simulink model "proyecto_2"  (R2021b)
settings: Solver=FixedStepDiscrete  StartTime=0.0  StopTime=Tsim  FixedStep=Tint  MaxStep=1e-6  RelTol=1e-6
InitFcn:
  | run init_fcn.m;
values from neighbouring files (symbols this model uses):
  C_init_v = 317    [init_fcn.m]
  C_load = 5e-2    (= 0.05)    [init_fcn.m]
  C_V = c_v * ro_air * volume_room    (= 220.63309632)    [init_fcn.m]
  Irr = 1000    [init_fcn.m]
  K_cond = Window_area * k_glass / esp    (= 158.4)    [init_fcn.m]
  L_s = 5e-3    (= 0.005)    [init_fcn.m]
  R_cuarto = 100    [init_fcn.m]
  shift = (180/3)/360 * Ts    (= 8.33333333333e-05)    [init_fcn.m]
  ss2 = c2d(ss2c, T_pred, 'tustin')    [init_fcn.m]
  T_ext = 15    [init_fcn.m]
  T_pred = Ts    (= 0.0005)    [init_fcn.m]
  Tint = 5e-5    (= 5e-05)    [init_fcn.m]
  Ts = 0.0005    [init_fcn.m]
  V_H4 = 300    [init_fcn.m]
  V_source = 230 * sqrt(2)    [init_fcn.m]
undefined symbols (not defined in the file or in its folder): DiscIntNeverNeededParam, F, K, Kobs, M, N, N2, Q, T_Enable, Temp_ref, Tsim, U0, X0
libraries: spsIGBTDiodeLib x17, spsVoltageMeasurementLib x11, simulink x8, spsCurrentMeasurementLib x8, slpidlib x6, spsSeriesRLCBranchLib x5, spsParallelRLCBranchLib x4, spsPVArrayLib x3, spsACVoltageSourceLib x1, spsDiodeLib x1, spspowerguiLib x1
(part 1 of 2)
settings Model: Creator=david  LastModifiedBy=david
settings DebuggingCC: UnderSpecifiedDimensionMsg=warning

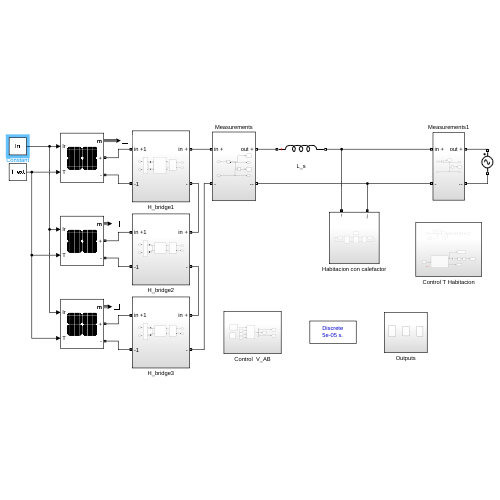
[thumbnail: Simulink's stored preview of the top-level diagram]
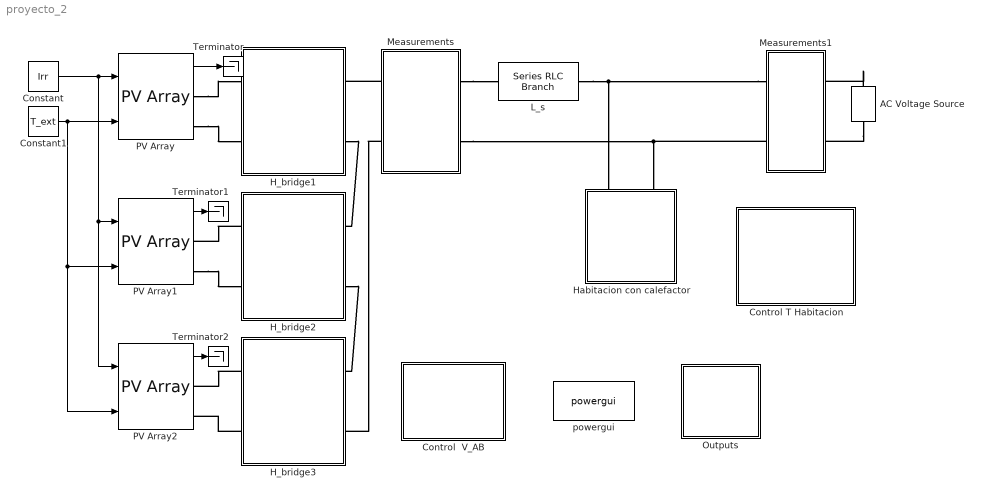
== system proyecto_2 ==
  AC Voltage Source : spsACVoltageSourceLib/AC Voltage Source  Amplitude=V_source  Phase=0  Frequency=50  SampleTime=0  Measurements=None  BusType=swing  Pref=10e3  Qref=0  Qmin=-inf  Qmax=+inf
  Constant : Constant  Value=Irr
  Constant1 : Constant  Value=T_ext
  Control  V_AB : Subsystem
  Control T Habitacion : Subsystem
  H_bridge1 : Subsystem
  H_bridge2 : Subsystem
  H_bridge3 : Subsystem
  Habitacion con calefactor : Subsystem
  L_s : spsSeriesRLCBranchLib/Series RLC Branch  LConnTagsString=__new0  RConnTagsString=__new0  BranchType=L  Resistance=1  Inductance=L_s*5  SetiL0=off  InitialCurrent=0  Capacitance=1e-6  Setx0=off  InitialVoltage=0  Measurements=None
  Measurements : Subsystem
  Measurements1 : Subsystem
  Outputs : Subsystem
  PV Array : spsPVArrayLib/PV Array  Npar=1  Nser=10  PlotType=array @ 1000 W/m2 & specified temperatures  S_vec="[ 1000  500  100 ]"  Temp_C_vec="[ 45 25  ]"  ModuleName=Ablytek 6PN6A230-A0  PlotWhenSelected=off  Pm=230.1288  Ncell=60  Voc=36.42  Isc=8.1  Vm=30.36  Im=7.58  beta_Voc_pc=-0.359  alpha_Isc_pc=0.097  beta_Voc=-0.13075  alpha_Isc=0.007857  IL=8.1068  I0=2.7914e-10  nI=0.98144  Rsh=234.4444  Rs=0.19819  RobustModel=off  RobustCellTemperature=313.3991  BAL=on  Tc=1e-6  Tfilter=5e-5
  PV Array1 : spsPVArrayLib/PV Array  Npar=1  Nser=10  PlotType=array @ 1000 W/m2 & specified temperatures  S_vec="[ 1000  500  100 ]"  Temp_C_vec="[ 45 25  ]"  ModuleName=Ablytek 6PN6A230-A0  PlotWhenSelected=off  Pm=230.1288  Ncell=60  Voc=36.42  Isc=8.1  Vm=30.36  Im=7.58  beta_Voc_pc=-0.359  alpha_Isc_pc=0.097  beta_Voc=-0.13075  alpha_Isc=0.007857  IL=8.1068  I0=2.7914e-10  nI=0.98144  Rsh=234.4444  Rs=0.19819  RobustModel=off  RobustCellTemperature=313.3991  BAL=on  Tc=1e-6  Tfilter=5e-5
  PV Array2 : spsPVArrayLib/PV Array  Npar=1  Nser=10  PlotType=array @ 1000 W/m2 & specified temperatures  S_vec="[ 1000  500  100 ]"  Temp_C_vec="[ 45 25  ]"  ModuleName=Ablytek 6PN6A230-A0  PlotWhenSelected=off  Pm=230.1288  Ncell=60  Voc=36.42  Isc=8.1  Vm=30.36  Im=7.58  beta_Voc_pc=-0.359  alpha_Isc_pc=0.097  beta_Voc=-0.13075  alpha_Isc=0.007857  IL=8.1068  I0=2.7914e-10  nI=0.98144  Rsh=234.4444  Rs=0.19819  RobustModel=off  RobustCellTemperature=313.3991  BAL=on  Tc=1e-6  Tfilter=5e-5
  Terminator : Terminator
  Terminator1 : Terminator
  Terminator2 : Terminator
  powergui : spspowerguiLib/powergui  Priority=1  SimulationMode=Discrete  SampleTime=Tint  frequency=60  Iterations=50  frequencyindice=0  Pbase=100e6  ErrMax=1e-4  UnitsV=kV  UnitsW=MW  buscounter=0  FunctionMessages=off  echomessages=off  EnableUseOfTLC=off  CurrentSourceSwitches=off  DisableSnubberDevices=off  DisableRonSwitches=off  DisableVfSwitches=off  DisplayEquations=off  AutomaticDiscreteSolvers=off  SolverType=Tustin/Backward Euler (TBE)  Interpol=off  ExternalGateDelay=off  methode=off  Ts=100  x0status=blocks  SPID=on  SwTol=0  HookPort=off  NonlinearTolerance=1e-4  nMaxIteration=100  ContinueOnMaxIteration=off  RestoreLinks=warning  ResistiveCurrentMeasurement=off  Frange=[0:2:500]  Ylog=off  Xlog=on  ShowGrid=off  save=off  variable=ZData  structure=0  ZoomFFT=off  StartTime=0.0  cycles=1  DisplayStyle=1  fundamental=60  FreqAxis=off  MaxFrequency=1000  frequencyindicesteady=1  RmsSteady=1  display=off
  wires:
  Constant1/1 -> PV Array1/2, PV Array2/2, PV Array/2
  Constant/1 -> PV Array2/1, PV Array1/1, PV Array/1
  PV Array/1 -> Terminator/1
  PV Array1/1 -> Terminator1/1
  PV Array2/1 -> Terminator2/1
  connections:
  PV Array/RConn2 -- H_bridge1/LConn2
  PV Array/RConn1 -- H_bridge1/LConn1
  Measurements/LConn1 -- H_bridge1/RConn1
  Measurements/RConn1 -- L_s/LConn1
  Measurements1/LConn2 -- Measurements/RConn2 -- Habitacion con calefactor/LConn2
  AC Voltage Source/RConn1 -- Measurements1/RConn1
  AC Voltage Source/LConn1 -- Measurements1/RConn2
  H_bridge1/RConn2 -- H_bridge2/RConn1
  H_bridge3/LConn1 -- PV Array2/RConn1
  H_bridge2/RConn2 -- H_bridge3/RConn1
  Measurements/LConn2 -- H_bridge3/RConn2
  PV Array1/RConn2 -- H_bridge2/LConn2
  H_bridge2/LConn1 -- PV Array1/RConn1
  H_bridge3/LConn2 -- PV Array2/RConn2
  L_s/RConn1 -- Measurements1/LConn1 -- Habitacion con calefactor/LConn1

== system proyecto_2/Control  V_AB ==
  DC-bus control : Subsystem
  Demux1 : Demux  Outputs=3
  S-Function : S-Function  FunctionName=ff3dm  SFunctionDeploymentMode=off  EnableBusSupport=off
  reassignment : Subsystem
  tag scope: d_1=global, d_2=global, d_3=global
  wires:
  [I_ab] -> S-Function/2
  Demux1/1 -> [d_1]
  Demux1/2 -> [d_2]
  Demux1/3 -> [d_3]
  S-Function/1 -> Demux1/1
  [refs] -> S-Function/4
  [V_dcH] -> S-Function/3
  DC-bus control/1(Out1) -> S-Function/1

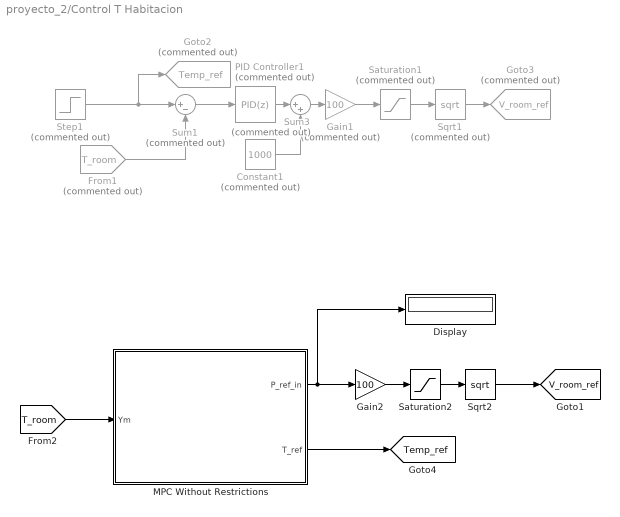
== system proyecto_2/Control T Habitacion ==
  Constant1 : Constant  Commented=on  Value=1000
  Display : Display
  From1 : From  Commented=on  GotoTag=T_room  TagVisibility=global
  Gain1 : Gain  Commented=on  Gain=100
  Gain2 : Gain  Gain=100
  Goto2 : Goto  Commented=on  GotoTag=Temp_ref  TagVisibility=global
  Goto3 : Goto  Commented=on  GotoTag=V_room_ref  TagVisibility=global
  MPC Without Restrictions : Subsystem
  PID Controller1 : slpidlib/PID Controller  Commented=on  Controller=PID  Form=Parallel  TimeDomain=Discrete-time  UseExternalTs=off  SampleTime=10*Ts  IntegratorMethod=Forward Euler  FilterMethod=Forward Euler  ControllerParametersSource=internal  P=200  I=500  D=0  UseFilter=on  N=100  TunerSelectOption=Transfer Function Based (PID Tuner App)  InitialConditionSource=internal  InitialConditionForIntegrator=0  InitialConditionForFilter=0  DifferentiatorICPrevScaledInput=0  ExternalReset=none  TrackingMode=off  Kt=1  LimitOutput=off  SatLimitsSource=internal  UpperSaturationLimit=inf  LowerSaturationLimit=-inf  LinearizeAsGain=on  AntiWindupMode=none  Kb=1  POutMin=[]  POutMax=[]  IOutMin=[]  IOutMax=[]  DOutMin=[]  DOutMax=[]  NOutMin=[]  NOutMax=[]  SumOutMin=[]  SumOutMax=[]  SaturationOutMin=[]  SaturationOutMax=[]  PParamMin=[]  PParamMax=[]  IParamMin=[]  IParamMax=[]  DParamMin=[]  DParamMax=[]  NParamMin=[]  NParamMax=[]  KbParamMin=[]  KbParamMax=[]  KtParamMin=[]  KtParamMax=[]  KbOutMin=[]  KbOutMax=[]  KtOutMin=[]  KtOutMax=[]  IntegratorOutMin=[]  IntegratorOutMax=[]  FilterOutMin=[]  FilterOutMax=[]  SumI1OutMin=[]  SumI1OutMax=[]  SumI2OutMin=[]  SumI2OutMax=[]  SumI3OutMin=[]  SumI3OutMax=[]  SumI4OutMin=[]  SumI4OutMax=[]  SumDOutMin=[]  SumDOutMax=[]  DifferentiatorOutMin=[]  DifferentiatorOutMax=[]  FilterDiffOutCoefMin=[]  FilterDiffOutCoefMax=[]  ReciprocalOutMin=[]  ReciprocalOutMax=[]  SumDenOutMin=[]  SumDenOutMax=[]  SumNumOutMin=[]  SumNumOutMax=[]  DivideOutMin=[]  DivideOutMax=[]  UdiffTsProdOutMin=[]  UdiffTsProdOutMax=[]  NTsProdOutMin=[]  NTsProdOutMax=[]  UintegralTsProdOutMin=[]  UintegralTsProdOutMax=[]  UngainTsProdOutMin=[]  UngainTsProdOutMax=[]  IntegratorContinuousStateAttributes=''  IntegratorStateMustResolveToSignalObject=off  IntegratorRTWStateStorageClass=Auto  FilterContinuousStateAttributes=''  FilterStateMustResolveToSignalObject=off  FilterRTWStateStorageClass=Auto  ParallelPVariant=InternalParameters  IdealPVariant=Disabled  IVariant=InternalParameters  DVariant=InternalParameters  IntegratorVariant=Discrete  SatVariant=Disabled  AWVariant=Passthrough  PCopyVariant=Disabled  TRVariant=Disabled  FdbkBlocksVariant=Forward  IdealPFdbkVariant=Disabled  SatFdbkVariant=Disabled  DerivativeFilterVariant=ForwardEulerFilter  NVariant=InternalParameters  NCopyVariant=Disabled  FilterICVariant=InternalICsFilter  IntegratorICVariant=InternalICs  ExternalResetVariant=Disabled  TRSumVariant=Passthrough  SumFdbkVariant=Disabled  SumVariant=Sum_PID  TsampFilterVariant=InternalTs  TsampNgainVariant=Passthrough  TsampIntegralVariant=Passthrough  ExternalSaturationOutDataTypeStr=Inherit: Same as second input
  Saturation1 : Saturate  Commented=on  UpperLimit=inf  LowerLimit=0
  Saturation2 : Saturate  UpperLimit=inf  LowerLimit=0
  Sqrt1 : Sqrt  Commented=on  SaturateOnIntegerOverflow=on
  Sqrt2 : Sqrt  SaturateOnIntegerOverflow=on
  Step1 : Step  Commented=on  Time=5  Before=20  After=25  SampleTime=0
  Sum1 : Sum  Commented=on  Inputs=|+-
  Sum3 : Sum  Commented=on  Inputs=|++
  tag scope: Temp_ref=global, V_room_ref=global
  wires:
  PID Controller1/1 -> Sum3/1
  Sum1/1 -> PID Controller1/1
  Constant1/1 -> Sum3/2
  Sqrt1/1 -> Goto3/1
  Gain1/1 -> Saturation1/1
  From1/1 -> Sum1/2
  Saturation1/1 -> Sqrt1/1
  Sum3/1 -> Gain1/1
  Step1/1 -> Goto2/1, Sum1/1
  Saturation2/1 -> Sqrt2/1
  Gain2/1 -> Saturation2/1
  MPC Without Restrictions/2(T_ref) -> [Temp_ref]
  MPC Without Restrictions/1(P_ref_in) -> Gain2/1, Display/1
  Sqrt2/1 -> [V_room_ref]
  [T_room] -> MPC Without Restrictions/1(Ym)
  ? -> ?

== system proyecto_2/H_bridge1 ==
  H_basic : Subsystem
  Measurements : Subsystem
  Measurements1 : Subsystem
  Parallel RLC Branch : spsParallelRLCBranchLib/Parallel RLC Branch  LConnTagsString=a  RConnTagsString=__new0  BranchType=C  Resistance=1  Inductance=1e-3  SetiL0=off  InitialCurrent=0  Capacitance=C_load  Setx0=on  InitialVoltage=C_init_v  Measurements=None
  in +1 : PMIOPort  Side=Left
  -1 : PMIOPort  Port=2  Side=Left
  in + : PMIOPort  Port=3  Side=Right
  - : PMIOPort  Port=4  Side=Right
  connections:
  Measurements1/RConn1 -- Parallel RLC Branch/LConn1 -- H_basic/LConn1
  Measurements/LConn1 -- in +/RConn1
  Measurements1/RConn2 -- Parallel RLC Branch/RConn1 -- H_basic/LConn2
  Measurements1/LConn1 -- in +1/RConn1
  Measurements1/LConn2 -- -1/RConn1
  Measurements/RConn2 -- H_basic/RConn2
  Measurements/LConn2 -- -/RConn1
  Measurements/RConn1 -- H_basic/RConn1

== system proyecto_2/H_bridge2 ==
  H_basic : Subsystem
  Measurements : Subsystem
  Measurements1 : Subsystem
  Parallel RLC Branch : spsParallelRLCBranchLib/Parallel RLC Branch  LConnTagsString=a  RConnTagsString=__new0  BranchType=C  Resistance=1  Inductance=1e-3  SetiL0=off  InitialCurrent=0  Capacitance=C_load  Setx0=on  InitialVoltage=C_init_v  Measurements=None
  in +1 : PMIOPort  Side=Left
  -1 : PMIOPort  Port=2  Side=Left
  in + : PMIOPort  Port=3  Side=Right
  - : PMIOPort  Port=4  Side=Right
  connections:
  Measurements1/RConn1 -- Parallel RLC Branch/LConn1 -- H_basic/LConn1
  Measurements/LConn1 -- in +/RConn1
  Measurements1/RConn2 -- Parallel RLC Branch/RConn1 -- H_basic/LConn2
  Measurements1/LConn1 -- in +1/RConn1
  Measurements1/LConn2 -- -1/RConn1
  H_basic/RConn2 -- Measurements/RConn2
  Measurements/LConn2 -- -/RConn1
  H_basic/RConn1 -- Measurements/RConn1

== system proyecto_2/H_bridge3 ==
  H_basic : Subsystem
  Measurements : Subsystem
  Measurements1 : Subsystem
  Parallel RLC Branch : spsParallelRLCBranchLib/Parallel RLC Branch  LConnTagsString=a  RConnTagsString=__new0  BranchType=C  Resistance=1  Inductance=1e-3  SetiL0=off  InitialCurrent=0  Capacitance=C_load  Setx0=on  InitialVoltage=C_init_v  Measurements=None
  in +1 : PMIOPort  Side=Left
  -1 : PMIOPort  Port=2  Side=Left
  in + : PMIOPort  Port=3  Side=Right
  - : PMIOPort  Port=4  Side=Right
  connections:
  Measurements1/RConn1 -- Parallel RLC Branch/LConn1 -- H_basic/LConn1
  Measurements/LConn1 -- in +/RConn1
  Measurements1/RConn2 -- H_basic/LConn2 -- Parallel RLC Branch/RConn1
  Measurements1/LConn1 -- in +1/RConn1
  Measurements1/LConn2 -- -1/RConn1
  H_basic/RConn2 -- Measurements/RConn2
  Measurements/LConn2 -- -/RConn1
  H_basic/RConn1 -- Measurements/RConn1

== system proyecto_2/Habitacion con calefactor ==
  Buck-Boost : Subsystem
  H_bridge4 : Subsystem
  L_s : spsSeriesRLCBranchLib/Series RLC Branch  LConnTagsString=__new0  RConnTagsString=__new0  BranchType=L  Resistance=1  Inductance=L_s  SetiL0=off  InitialCurrent=0  Capacitance=1e-6  Setx0=off  InitialVoltage=0  Measurements=None
  Measurements : Subsystem
  Room : Subsystem
  Series RLC Branch : spsSeriesRLCBranchLib/Series RLC Branch  LConnTagsString=__new0  RConnTagsString=__new0  BranchType=R  Resistance=R_cuarto  Inductance=1e-3  SetiL0=off  InitialCurrent=0  Capacitance=1e-6  Setx0=off  InitialVoltage=0  Measurements=None
  ~ : PMIOPort  Side=Left
  ~- : PMIOPort  Port=2  Side=Left
  connections:
  ~-/RConn1 -- H_bridge4/RConn2
  L_s/LConn1 -- H_bridge4/RConn1
  L_s/RConn1 -- ~/RConn1
  Measurements/RConn1 -- Series RLC Branch/LConn1
  Series RLC Branch/RConn1 -- Measurements/RConn2
  Buck-Boost/RConn1 -- Measurements/LConn1
  Measurements/LConn2 -- Buck-Boost/RConn2
  Buck-Boost/LConn2 -- H_bridge4/LConn2
  Buck-Boost/LConn1 -- H_bridge4/LConn1

== system proyecto_2/Measurements ==
  I : spsCurrentMeasurementLib/Current Measurement  PhasorSimulation=off  OutputType=Complex  PSBequivalent=0
  V : spsVoltageMeasurementLib/Voltage Measurement  PhasorSimulation=off  OutputType=Complex  PSBequivalent=0
  in + : PMIOPort  Side=Left
  - : PMIOPort  Port=2  Side=Left
  out + : PMIOPort  Port=3  Side=Right
  -- : PMIOPort  Port=4  Side=Right
  tag scope: I_ab=global, V_s=global
  wires:
  V/1 -> [V_s]
  I/1 -> [I_ab]
  connections:
  V/LConn2 -- --/RConn1 -- -/RConn1
  out +/RConn1 -- V/LConn1 -- I/RConn1
  in +/RConn1 -- I/LConn1

== system proyecto_2/Measurements1 ==
  Current Measurement : spsCurrentMeasurementLib/Current Measurement  PhasorSimulation=off  OutputType=Complex  PSBequivalent=0
  V : spsVoltageMeasurementLib/Voltage Measurement  PhasorSimulation=off  OutputType=Complex  PSBequivalent=0
  in + : PMIOPort  Side=Left
  - : PMIOPort  Port=2  Side=Left
  out + : PMIOPort  Port=3  Side=Right
  -- : PMIOPort  Port=4  Side=Right
  tag scope: I_grid=global, V_grid=global
  wires:
  V/1 -> [V_grid]
  Current Measurement/1 -> [I_grid]
  connections:
  V/LConn2 -- --/RConn1 -- -/RConn1
  V/LConn1 -- Current Measurement/RConn1 -- out +/RConn1
  Current Measurement/LConn1 -- in +/RConn1

== system proyecto_2/Outputs ==
  Habitacion : Subsystem
  Placas : Subsystem
  Resumen : Subsystem

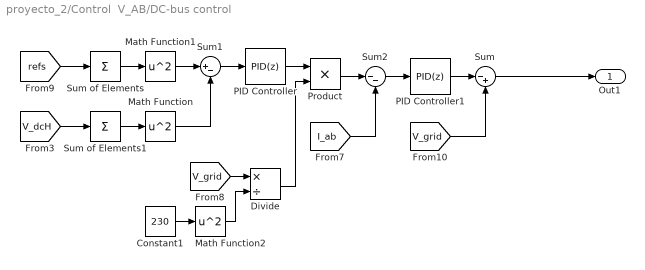
== system proyecto_2/Control  V_AB/DC-bus control ==
  Constant1 : Constant  Value=230
  Divide : Product  Inputs=*/
  Math Function : Math  Operator=square  SaturateOnIntegerOverflow=on
  Math Function1 : Math  Operator=square  SaturateOnIntegerOverflow=on
  Math Function2 : Math  Operator=square  SaturateOnIntegerOverflow=on
  PID Controller : slpidlib/PID Controller  Controller=PID  Form=Parallel  TimeDomain=Discrete-time  UseExternalTs=off  SampleTime=Ts  IntegratorMethod=Forward Euler  FilterMethod=Forward Euler  ControllerParametersSource=internal  P=3  I=10  D=0  UseFilter=on  N=100  TunerSelectOption=Transfer Function Based (PID Tuner App)  InitialConditionSource=internal  InitialConditionForIntegrator=0  InitialConditionForFilter=0  DifferentiatorICPrevScaledInput=0  ExternalReset=none  TrackingMode=off  Kt=1  LimitOutput=off  SatLimitsSource=internal  UpperSaturationLimit=inf  LowerSaturationLimit=-inf  LinearizeAsGain=on  AntiWindupMode=none  Kb=1  POutMin=[]  POutMax=[]  IOutMin=[]  IOutMax=[]  DOutMin=[]  DOutMax=[]  NOutMin=[]  NOutMax=[]  SumOutMin=[]  SumOutMax=[]  SaturationOutMin=[]  SaturationOutMax=[]  PParamMin=[]  PParamMax=[]  IParamMin=[]  IParamMax=[]  DParamMin=[]  DParamMax=[]  NParamMin=[]  NParamMax=[]  KbParamMin=[]  KbParamMax=[]  KtParamMin=[]  KtParamMax=[]  KbOutMin=[]  KbOutMax=[]  KtOutMin=[]  KtOutMax=[]  IntegratorOutMin=[]  IntegratorOutMax=[]  FilterOutMin=[]  FilterOutMax=[]  SumI1OutMin=[]  SumI1OutMax=[]  SumI2OutMin=[]  SumI2OutMax=[]  SumI3OutMin=[]  SumI3OutMax=[]  SumI4OutMin=[]  SumI4OutMax=[]  SumDOutMin=[]  SumDOutMax=[]  DifferentiatorOutMin=[]  DifferentiatorOutMax=[]  FilterDiffOutCoefMin=[]  FilterDiffOutCoefMax=[]  ReciprocalOutMin=[]  ReciprocalOutMax=[]  SumDenOutMin=[]  SumDenOutMax=[]  SumNumOutMin=[]  SumNumOutMax=[]  DivideOutMin=[]  DivideOutMax=[]  UdiffTsProdOutMin=[]  UdiffTsProdOutMax=[]  NTsProdOutMin=[]  NTsProdOutMax=[]  UintegralTsProdOutMin=[]  UintegralTsProdOutMax=[]  UngainTsProdOutMin=[]  UngainTsProdOutMax=[]  IntegratorContinuousStateAttributes=''  IntegratorStateMustResolveToSignalObject=off  IntegratorRTWStateStorageClass=Auto  FilterContinuousStateAttributes=''  FilterStateMustResolveToSignalObject=off  FilterRTWStateStorageClass=Auto  ParallelPVariant=InternalParameters  IdealPVariant=Disabled  IVariant=InternalParameters  DVariant=InternalParameters  IntegratorVariant=Discrete  SatVariant=Disabled  AWVariant=Passthrough  PCopyVariant=Disabled  TRVariant=Disabled  FdbkBlocksVariant=Forward  IdealPFdbkVariant=Disabled  SatFdbkVariant=Disabled  DerivativeFilterVariant=ForwardEulerFilter  NVariant=InternalParameters  NCopyVariant=Disabled  FilterICVariant=InternalICsFilter  IntegratorICVariant=InternalICs  ExternalResetVariant=Disabled  TRSumVariant=Passthrough  SumFdbkVariant=Disabled  SumVariant=Sum_PID  TsampFilterVariant=InternalTs  TsampNgainVariant=Passthrough  TsampIntegralVariant=Passthrough  ExternalSaturationOutDataTypeStr=Inherit: Same as second input
  PID Controller1 : slpidlib/PID Controller  Controller=PID  Form=Parallel  TimeDomain=Discrete-time  UseExternalTs=off  SampleTime=Ts  IntegratorMethod=Forward Euler  FilterMethod=Forward Euler  ControllerParametersSource=internal  P=5  I=10  D=0  UseFilter=on  N=100  TunerSelectOption=Transfer Function Based (PID Tuner App)  InitialConditionSource=internal  InitialConditionForIntegrator=0  InitialConditionForFilter=0  DifferentiatorICPrevScaledInput=0  ExternalReset=none  TrackingMode=off  Kt=1  LimitOutput=off  SatLimitsSource=internal  UpperSaturationLimit=inf  LowerSaturationLimit=-inf  LinearizeAsGain=on  AntiWindupMode=none  Kb=1  POutMin=[]  POutMax=[]  IOutMin=[]  IOutMax=[]  DOutMin=[]  DOutMax=[]  NOutMin=[]  NOutMax=[]  SumOutMin=[]  SumOutMax=[]  SaturationOutMin=[]  SaturationOutMax=[]  PParamMin=[]  PParamMax=[]  IParamMin=[]  IParamMax=[]  DParamMin=[]  DParamMax=[]  NParamMin=[]  NParamMax=[]  KbParamMin=[]  KbParamMax=[]  KtParamMin=[]  KtParamMax=[]  KbOutMin=[]  KbOutMax=[]  KtOutMin=[]  KtOutMax=[]  IntegratorOutMin=[]  IntegratorOutMax=[]  FilterOutMin=[]  FilterOutMax=[]  SumI1OutMin=[]  SumI1OutMax=[]  SumI2OutMin=[]  SumI2OutMax=[]  SumI3OutMin=[]  SumI3OutMax=[]  SumI4OutMin=[]  SumI4OutMax=[]  SumDOutMin=[]  SumDOutMax=[]  DifferentiatorOutMin=[]  DifferentiatorOutMax=[]  FilterDiffOutCoefMin=[]  FilterDiffOutCoefMax=[]  ReciprocalOutMin=[]  ReciprocalOutMax=[]  SumDenOutMin=[]  SumDenOutMax=[]  SumNumOutMin=[]  SumNumOutMax=[]  DivideOutMin=[]  DivideOutMax=[]  UdiffTsProdOutMin=[]  UdiffTsProdOutMax=[]  NTsProdOutMin=[]  NTsProdOutMax=[]  UintegralTsProdOutMin=[]  UintegralTsProdOutMax=[]  UngainTsProdOutMin=[]  UngainTsProdOutMax=[]  IntegratorContinuousStateAttributes=''  IntegratorStateMustResolveToSignalObject=off  IntegratorRTWStateStorageClass=Auto  FilterContinuousStateAttributes=''  FilterStateMustResolveToSignalObject=off  FilterRTWStateStorageClass=Auto  ParallelPVariant=InternalParameters  IdealPVariant=Disabled  IVariant=InternalParameters  DVariant=InternalParameters  IntegratorVariant=Discrete  SatVariant=Disabled  AWVariant=Passthrough  PCopyVariant=Disabled  TRVariant=Disabled  FdbkBlocksVariant=Forward  IdealPFdbkVariant=Disabled  SatFdbkVariant=Disabled  DerivativeFilterVariant=ForwardEulerFilter  NVariant=InternalParameters  NCopyVariant=Disabled  FilterICVariant=InternalICsFilter  IntegratorICVariant=InternalICs  ExternalResetVariant=Disabled  TRSumVariant=Passthrough  SumFdbkVariant=Disabled  SumVariant=Sum_PID  TsampFilterVariant=InternalTs  TsampNgainVariant=Passthrough  TsampIntegralVariant=Passthrough  ExternalSaturationOutDataTypeStr=Inherit: Same as second input
  Product : Product
  Sum : Sum  Inputs=|-+
  Sum of Elements : Sum  Inputs=+
  Sum of Elements1 : Sum  Inputs=+
  Sum1 : Sum  Inputs=|+-
  Sum2 : Sum  Inputs=|--
  Out1 : Outport
  wires:
  [V_grid] -> Sum/2
  [I_ab] -> Sum2/2
  [V_dcH] -> Sum of Elements1/1
  Sum of Elements/1 -> Math Function1/1
  PID Controller1/1 -> Sum/1
  Product/1 -> Sum2/1
  Sum1/1 -> PID Controller/1
  Sum/1 -> Out1/1
  PID Controller/1 -> Product/1
  [refs] -> Sum of Elements/1
  Sum2/1 -> PID Controller1/1
  [V_grid] -> Divide/1
  Divide/1 -> Product/2
  Math Function1/1 -> Sum1/1
  Math Function2/1 -> Divide/2
  Math Function/1 -> Sum1/2
  Constant1/1 -> Math Function2/1
  Sum of Elements1/1 -> Math Function/1

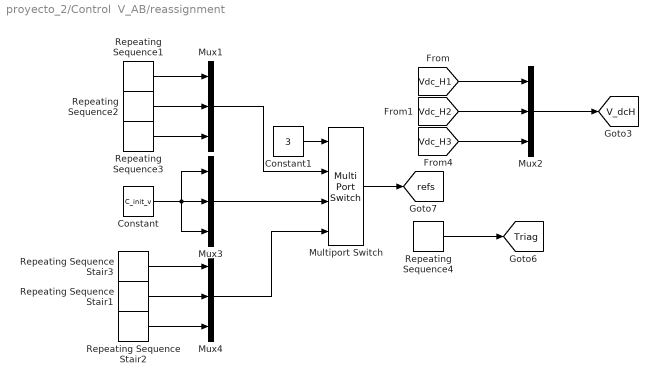
== system proyecto_2/Control  V_AB/reassignment ==
  Constant : Constant  Value=C_init_v
  Constant1 : Constant  Value=3
  Multiport Switch : MultiPortSwitch  DiagnosticForDefault=None
  Mux{1..4} (4 alike) : Mux  Inputs=3
  Repeating Sequence Stair1 : simulink/Sources/Repeating Sequence Stair  OutValues=[C_init_v, C_init_v-5 , C_init_v, C_init_v+5].'  tsamp=0.2  OutMin=[]  OutMax=[]  OutDataTypeStr=double  OutputDataTypeScalingMode=double  OutDataType=fixdt(0,8)  ConRadixGroup=Best Precision: Vector-wise  OutScaling=2^-12
  Repeating Sequence Stair2 : simulink/Sources/Repeating Sequence Stair  OutValues=[C_init_v+5, C_init_v , C_init_v-5, C_init_v].'  tsamp=0.2  OutMin=[]  OutMax=[]  OutDataTypeStr=double  OutputDataTypeScalingMode=double  OutDataType=fixdt(0,8)  ConRadixGroup=Best Precision: Vector-wise  OutScaling=2^-12
  Repeating Sequence Stair3 : simulink/Sources/Repeating Sequence Stair  OutValues=[C_init_v, C_init_v+5 , C_init_v, C_init_v-5].'  tsamp=0.2  OutMin=[]  OutMax=[]  OutDataTypeStr=double  OutputDataTypeScalingMode=double  OutDataType=fixdt(0,8)  ConRadixGroup=Best Precision: Vector-wise  OutScaling=2^-12
  Repeating Sequence1 : simulink/Sources/Repeating Sequence  rep_seq_t=[0 1 2 3 4 5 6 7 8 9 10]  rep_seq_y=[C_init_v C_init_v 350 350 250 250 300 300 330 330 C_init_v]
  Repeating Sequence2 : simulink/Sources/Repeating Sequence  rep_seq_t=[0 1 2 3 4 5 6 7 8 9 10]  rep_seq_y=[C_init_v C_init_v 250 250 350 350 320 320 300 300 C_init_v]
  Repeating Sequence3 : simulink/Sources/Repeating Sequence  rep_seq_t=[0 1 2 3 4 5 6 7 8 9 10]  rep_seq_y=[C_init_v C_init_v 330 330 280 280 270 270 280 280 C_init_v]
  Repeating Sequence4 : simulink/Sources/Repeating Sequence  rep_seq_t=[0 Ts/2 Ts]  rep_seq_y=[-1 1 -1]
  tag scope: Triag=global, V_dcH=global, refs=global
  wires:
  Repeating Sequence Stair3/1 -> Mux4/1
  [Vdc_H1] -> Mux2/1
  Mux2/1 -> [V_dcH]
  Mux1/1 -> Multiport Switch/2
  [Vdc_H3] -> Mux2/3
  Constant/1 -> Mux3/3, Mux3/1, Mux3/2
  Repeating Sequence3/1 -> Mux1/3
  Repeating Sequence1/1 -> Mux1/1
  Repeating Sequence Stair2/1 -> Mux4/3
  Constant1/1 -> Multiport Switch/1
  Repeating Sequence2/1 -> Mux1/2
  Repeating Sequence4/1 -> [Triag]
  Mux4/1 -> Multiport Switch/4
  [Vdc_H2] -> Mux2/2
  Repeating Sequence Stair1/1 -> Mux4/2
  Mux3/1 -> Multiport Switch/3
  Multiport Switch/1 -> [refs]

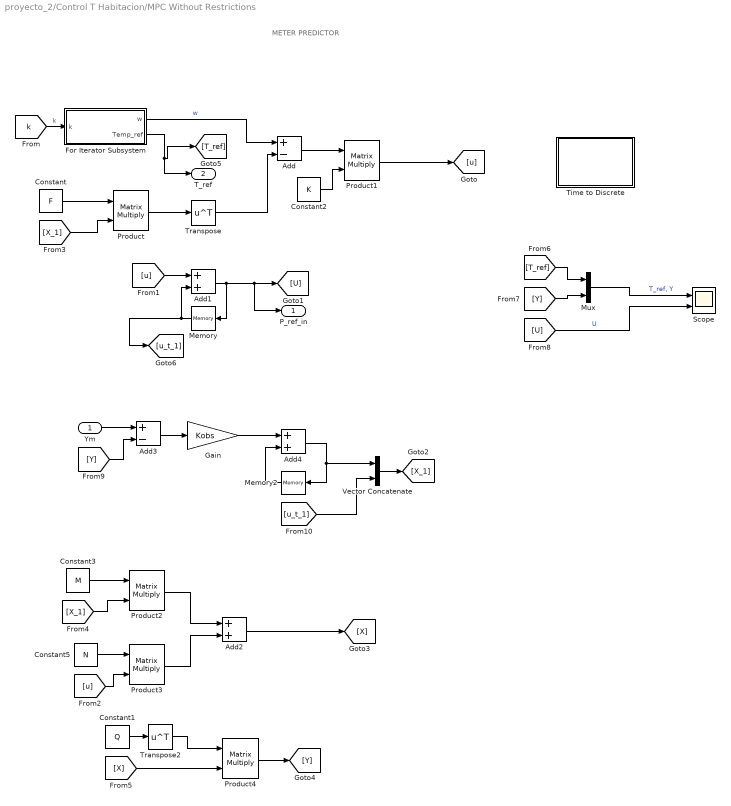
== system proyecto_2/Control T Habitacion/MPC Without Restrictions ==
  note: METER PREDICTOR
  Ym : Inport
  Add : Sum  Inputs=+-
  Add1 : Sum
  Add2 : Sum
  Add3 : Sum  Inputs=+-
  Add4 : Sum
  Constant : Constant  Value=F
  Constant1 : Constant  Value=Q
  Constant2 : Constant  Value=K
  Constant3 : Constant  Value=M
  Constant5 : Constant  Value=N
  For Iterator Subsystem : Subsystem  TreatAsAtomicUnit=on
  Gain : Gain  Gain=Kobs
  Memory : Memory  InitialCondition=U0
  Memory2 : Memory  InitialCondition=X0
  Mux : Mux  Inputs=2
  Product{,1..4} (5 alike) : Product  Multiplication=Matrix(*)
  Scope : Scope  NumInputPorts=2
  Time to Discrete : Subsystem
  Transpose : Math  Operator=transpose  SaturateOnIntegerOverflow=on
  Transpose2 : Math  Operator=transpose  SaturateOnIntegerOverflow=on
  Vector Concatenate : Concatenate
  P_ref_in : Outport
  T_ref : Outport  Port=2
  wires:
  Transpose2/1 -> Product4/1
  [u] -> Product3/2
  [u] -> Add1/1
  Memory/1 -> Add1/2, [u_t_1]
  Add2/1 -> [X]
  Transpose/1 -> Add/2
  Product/1 -> Transpose/1
  Constant5/1 -> Product3/1
  Product3/1 -> Add2/2
  Product2/1 -> Add2/1
  [X_1] -> Product2/2
  [X_1] -> Product/2
  Constant1/1 -> Transpose2/1
  Add/1 -> Product1/1
  For Iterator Subsystem/2(Temp_ref) -> [T_ref], T_ref/1
  Constant2/1 -> Product1/2
  [U] -> Scope/2  "U"
  [k] -> For Iterator Subsystem/1(k)  "k"
  For Iterator Subsystem/1(w) -> Add/1  "w"
  Constant3/1 -> Product2/1
  [T_ref] -> Mux/1
  [Y] -> Mux/2
  Constant/1 -> Product/1
  Mux/1 -> Scope/1  "T_ref, Y"
  Product4/1 -> [Y]
  Product1/1 -> [u]
  [X] -> Product4/2
  Add1/1 -> P_ref_in/1, [U], Memory/1
  Ym/1 -> Add3/1
  [Y] -> Add3/2
  Add3/1 -> Gain/1
  Gain/1 -> Add4/1
  Add4/1 -> Vector Concatenate/1, Memory2/1
  Memory2/1 -> Add4/2
  [u_t_1] -> Vector Concatenate/2
  Vector Concatenate/1 -> [X_1]

== system proyecto_2/H_bridge1/H_basic ==
  Demux : Demux
  IGBT/Diode{,1..3} (4 alike) : spsIGBTDiodeLib/IGBT//Diode  Ron=1e-3  Rs=1e5  Cs=inf  Measurements=off
  Modulator2 : Subsystem
  out + : PMIOPort  Side=Left
  out - : PMIOPort  Port=2  Side=Left
  in + : PMIOPort  Port=3  Side=Right
  in - : PMIOPort  Port=4  Side=Right
  wires:
  Demux/1 -> IGBT/Diode/1
  Demux/4 -> IGBT/Diode3/1
  Demux/2 -> IGBT/Diode2/1
  Demux/3 -> IGBT/Diode1/1
  Modulator2/1(Out1) -> Demux/1
  connections:
  IGBT/Diode2/RConn1 -- out -/RConn1 -- IGBT/Diode3/RConn1
  IGBT/Diode1/RConn1 -- in +/RConn1 -- IGBT/Diode3/LConn1
  IGBT/Diode/LConn1 -- out +/RConn1 -- IGBT/Diode1/LConn1
  IGBT/Diode/RConn1 -- in -/RConn1 -- IGBT/Diode2/LConn1

== system proyecto_2/H_bridge1/Measurements ==
  V : spsVoltageMeasurementLib/Voltage Measurement  PhasorSimulation=off  OutputType=Complex  PSBequivalent=0
  in + : PMIOPort  Side=Left
  - : PMIOPort  Port=2  Side=Left
  out + : PMIOPort  Port=3  Side=Right
  -- : PMIOPort  Port=4  Side=Right
  tag scope: Vac_H1=global
  wires:
  V/1 -> [Vac_H1]
  connections:
  V/LConn2 -- --/RConn1 -- -/RConn1
  V/LConn1 -- in +/RConn1 -- out +/RConn1

== system proyecto_2/H_bridge1/Measurements1 ==
  Current Measurement : spsCurrentMeasurementLib/Current Measurement  PhasorSimulation=off  OutputType=Complex  PSBequivalent=0
  V : spsVoltageMeasurementLib/Voltage Measurement  PhasorSimulation=off  OutputType=Complex  PSBequivalent=0
  in + : PMIOPort  Side=Left
  - : PMIOPort  Port=2  Side=Left
  out + : PMIOPort  Port=3  Side=Right
  -- : PMIOPort  Port=4  Side=Right
  tag scope: Idc_H1=global, Vdc_H1=global
  wires:
  V/1 -> [Vdc_H1]
  Current Measurement/1 -> [Idc_H1]
  connections:
  -/RConn1 -- V/LConn2 -- --/RConn1
  V/LConn1 -- Current Measurement/RConn1 -- out +/RConn1
  Current Measurement/LConn1 -- in +/RConn1

== system proyecto_2/H_bridge2/H_basic ==
  Demux : Demux
  IGBT/Diode{,1..3} (4 alike) : spsIGBTDiodeLib/IGBT//Diode  Ron=1e-3  Rs=1e5  Cs=inf  Measurements=off
  Modulator2 : Subsystem
  out + : PMIOPort  Side=Left
  out - : PMIOPort  Port=2  Side=Left
  in + : PMIOPort  Port=3  Side=Right
  in - : PMIOPort  Port=4  Side=Right
  wires:
  Demux/1 -> IGBT/Diode/1
  Demux/4 -> IGBT/Diode3/1
  Demux/2 -> IGBT/Diode2/1
  Demux/3 -> IGBT/Diode1/1
  Modulator2/1(Out1) -> Demux/1
  connections:
  IGBT/Diode2/RConn1 -- out -/RConn1 -- IGBT/Diode3/RConn1
  IGBT/Diode1/RConn1 -- in +/RConn1 -- IGBT/Diode3/LConn1
  IGBT/Diode/LConn1 -- out +/RConn1 -- IGBT/Diode1/LConn1
  IGBT/Diode/RConn1 -- in -/RConn1 -- IGBT/Diode2/LConn1

== system proyecto_2/H_bridge2/Measurements ==
  V : spsVoltageMeasurementLib/Voltage Measurement  PhasorSimulation=off  OutputType=Complex  PSBequivalent=0
  in + : PMIOPort  Side=Left
  - : PMIOPort  Port=2  Side=Left
  out + : PMIOPort  Port=3  Side=Right
  -- : PMIOPort  Port=4  Side=Right
  tag scope: Vac_H2=global
  wires:
  V/1 -> [Vac_H2]
  connections:
  V/LConn2 -- --/RConn1 -- -/RConn1
  V/LConn1 -- in +/RConn1 -- out +/RConn1

== system proyecto_2/H_bridge2/Measurements1 ==
  Current Measurement : spsCurrentMeasurementLib/Current Measurement  PhasorSimulation=off  OutputType=Complex  PSBequivalent=0
  V : spsVoltageMeasurementLib/Voltage Measurement  PhasorSimulation=off  OutputType=Complex  PSBequivalent=0
  in + : PMIOPort  Side=Left
  - : PMIOPort  Port=2  Side=Left
  out + : PMIOPort  Port=3  Side=Right
  -- : PMIOPort  Port=4  Side=Right
  tag scope: Idc_H2=global, Vdc_H2=global
  wires:
  V/1 -> [Vdc_H2]
  Current Measurement/1 -> [Idc_H2]
  connections:
  -/RConn1 -- V/LConn2 -- --/RConn1
  V/LConn1 -- out +/RConn1 -- Current Measurement/RConn1
  Current Measurement/LConn1 -- in +/RConn1

== system proyecto_2/H_bridge3/H_basic ==
  Demux : Demux
  IGBT/Diode{,1..3} (4 alike) : spsIGBTDiodeLib/IGBT//Diode  Ron=1e-3  Rs=1e5  Cs=inf  Measurements=off
  Modulator2 : Subsystem
  out + : PMIOPort  Side=Left
  out - : PMIOPort  Port=2  Side=Left
  in + : PMIOPort  Port=3  Side=Right
  in - : PMIOPort  Port=4  Side=Right
  wires:
  Demux/1 -> IGBT/Diode/1
  Demux/4 -> IGBT/Diode3/1
  Demux/2 -> IGBT/Diode2/1
  Demux/3 -> IGBT/Diode1/1
  Modulator2/1(Out1) -> Demux/1
  connections:
  IGBT/Diode2/RConn1 -- out -/RConn1 -- IGBT/Diode3/RConn1
  IGBT/Diode1/RConn1 -- in +/RConn1 -- IGBT/Diode3/LConn1
  IGBT/Diode/LConn1 -- out +/RConn1 -- IGBT/Diode1/LConn1
  IGBT/Diode/RConn1 -- in -/RConn1 -- IGBT/Diode2/LConn1

== system proyecto_2/H_bridge3/Measurements ==
  V : spsVoltageMeasurementLib/Voltage Measurement  PhasorSimulation=off  OutputType=Complex  PSBequivalent=0
  in + : PMIOPort  Side=Left
  - : PMIOPort  Port=2  Side=Left
  out + : PMIOPort  Port=3  Side=Right
  -- : PMIOPort  Port=4  Side=Right
  tag scope: Vac_H3=global
  wires:
  V/1 -> [Vac_H3]
  connections:
  V/LConn2 -- --/RConn1 -- -/RConn1
  V/LConn1 -- in +/RConn1 -- out +/RConn1

== system proyecto_2/H_bridge3/Measurements1 ==
  Current Measurement : spsCurrentMeasurementLib/Current Measurement  PhasorSimulation=off  OutputType=Complex  PSBequivalent=0
  V : spsVoltageMeasurementLib/Voltage Measurement  PhasorSimulation=off  OutputType=Complex  PSBequivalent=0
  in + : PMIOPort  Side=Left
  - : PMIOPort  Port=2  Side=Left
  out + : PMIOPort  Port=3  Side=Right
  -- : PMIOPort  Port=4  Side=Right
  tag scope: Idc_H3=global, Vdc_H3=global
  wires:
  V/1 -> [Vdc_H3]
  Current Measurement/1 -> [Idc_H3]
  connections:
  -/RConn1 -- V/LConn2 -- --/RConn1
  V/LConn1 -- out +/RConn1 -- Current Measurement/RConn1
  Current Measurement/LConn1 -- in +/RConn1

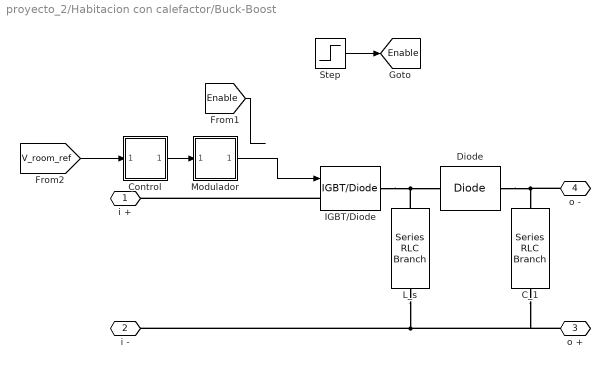
== system proyecto_2/Habitacion con calefactor/Buck-Boost ==
  C_1 : spsSeriesRLCBranchLib/Series RLC Branch  LConnTagsString=__new0  RConnTagsString=__new0  BranchType=C  Resistance=1  Inductance=L_s/2  SetiL0=off  InitialCurrent=0  Capacitance=C_load/10  Setx0=off  InitialVoltage=300  Measurements=None
  Control : Subsystem
  Diode : spsDiodeLib/Diode  Ron=1e-3  Lon=0  Vf=0.8  IC=0  UseSnubber=0  Rs=inf  Cs=250e-9  Measurements=off
  IGBT/Diode : spsIGBTDiodeLib/IGBT//Diode  Ron=1e-3  Rs=1e5  Cs=inf  Measurements=off
  L_s : spsSeriesRLCBranchLib/Series RLC Branch  LConnTagsString=__new0  RConnTagsString=__new0  BranchType=L  Resistance=1  Inductance=L_s * 12  SetiL0=off  InitialCurrent=0  Capacitance=1e-6  Setx0=off  InitialVoltage=0  Measurements=None
  Modulador : Subsystem
  Step : Step  Time=T_Enable  SampleTime=0
  i + : PMIOPort  Side=Left
  i - : PMIOPort  Port=2  Side=Left
  o + : PMIOPort  Port=3  Side=Right
  o - : PMIOPort  Port=4  Side=Right
  tag scope: Enable=global
  wires:
  Control/1(Out1) -> Modulador/1(In1)
  [V_room_ref] -> Control/1(In1)
  Step/1 -> [Enable]
  Modulador/1(Out1) -> IGBT/Diode/1
  [Enable] -> ?
  connections:
  L_s/LConn1 -- i -/RConn1 -- o +/RConn1 -- C_1/LConn1
  IGBT/Diode/RConn1 -- L_s/RConn1 -- Diode/RConn1
  o -/RConn1 -- C_1/RConn1 -- Diode/LConn1
  IGBT/Diode/LConn1 -- i +/RConn1

== system proyecto_2/Habitacion con calefactor/H_bridge4 ==
  H_basic : Subsystem
  Internal control : Subsystem
  Measurements : Subsystem
  Measurements1 : Subsystem
  Parallel RLC Branch : spsParallelRLCBranchLib/Parallel RLC Branch  LConnTagsString=a  RConnTagsString=__new0  BranchType=C  Resistance=1  Inductance=1e-3  SetiL0=off  InitialCurrent=0  Capacitance=C_load  Setx0=on  InitialVoltage=C_init_v  Measurements=None
  + : PMIOPort  Side=Left
  - : PMIOPort  Port=2  Side=Left
  ~+ : PMIOPort  Port=3  Side=Right
  ~- : PMIOPort  Port=4  Side=Right
  connections:
  Measurements1/RConn1 -- Parallel RLC Branch/LConn1 -- H_basic/LConn1
  Measurements/LConn1 -- ~+/RConn1
  Measurements1/RConn2 -- Parallel RLC Branch/RConn1 -- H_basic/LConn2
  Measurements1/LConn1 -- +/RConn1
  Measurements1/LConn2 -- -/RConn1
  H_basic/RConn2 -- Measurements/RConn2
  Measurements/LConn2 -- ~-/RConn1
  H_basic/RConn1 -- Measurements/RConn1

== system proyecto_2/Habitacion con calefactor/Measurements ==
  Current Measurement : spsCurrentMeasurementLib/Current Measurement  PhasorSimulation=off  OutputType=Complex  PSBequivalent=0
  V : spsVoltageMeasurementLib/Voltage Measurement  PhasorSimulation=off  OutputType=Complex  PSBequivalent=0
  in + : PMIOPort  Side=Left
  - : PMIOPort  Port=2  Side=Left
  out + : PMIOPort  Port=3  Side=Right
  -- : PMIOPort  Port=4  Side=Right
  tag scope: I_room=global, V_room=global
  wires:
  V/1 -> [V_room]
  Current Measurement/1 -> [I_room]
  connections:
  V/LConn2 -- --/RConn1 -- -/RConn1
  V/LConn1 -- Current Measurement/RConn1 -- out +/RConn1
  Current Measurement/LConn1 -- in +/RConn1

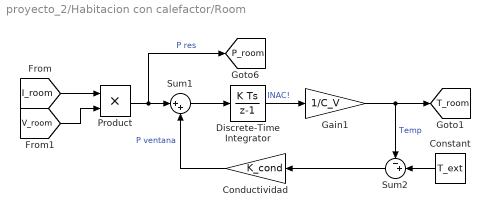
== system proyecto_2/Habitacion con calefactor/Room ==
  Conductividad : Gain  Gain=K_cond
  Constant : Constant  Value=T_ext
  Discrete-Time Integrator : DiscreteIntegrator  InitialCondition=T_ext * C_V  SampleTime=Tint  ICPrevOutput=DiscIntNeverNeededParam  ICPrevScaledInput=DiscIntNeverNeededParam
  Gain1 : Gain  Gain=1/C_V
  Product : Product
  Sum1 : Sum  Inputs=|++
  Sum2 : Sum  Inputs=-+|
  tag scope: P_room=global, T_room=global
  wires:
  Sum1/1 -> Discrete-Time Integrator/1
  Discrete-Time Integrator/1 -> Gain1/1  "INAC!"
  Gain1/1 -> [T_room], Sum2/1  "Temp"
  Conductividad/1 -> Sum1/2  "P ventana"
  Sum2/1 -> Conductividad/1
  Product/1 -> [P_room], Sum1/1  "P res"
  Constant/1 -> Sum2/2
  [V_room] -> Product/2
  [I_room] -> Product/1

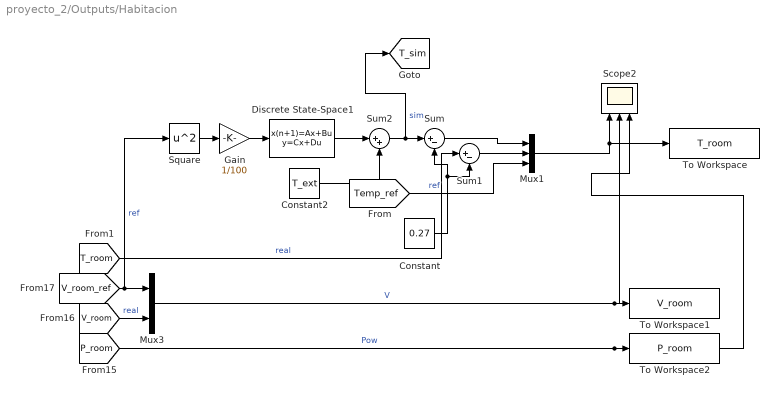
== system proyecto_2/Outputs/Habitacion ==
  Constant : Constant  Value=0.27
  Constant2 : Constant  Value=T_ext
  Discrete State-Space1 : DiscreteStateSpace  A=ss2.A  B=ss2.B  C=ss2.C  D=ss2.D  SampleTime=T_pred
  Gain : Gain  Gain=1/100
  Mux1 : Mux  Inputs=3
  Mux3 : Mux  Inputs=2
  Scope2 : Scope  NumInputPorts=3
  Square : Math  Operator=square  SaturateOnIntegerOverflow=on
  Sum : Sum  Inputs=|+-
  Sum1 : Sum  Inputs=|+-
  Sum2 : Sum  Inputs=|++
  To Workspace : ToWorkspace  VariableName=T_room  SaveFormat=Structure With Time  SampleTime=-1
  To Workspace1 : ToWorkspace  VariableName=V_room  SaveFormat=Structure With Time  SampleTime=-1
  To Workspace2 : ToWorkspace  VariableName=P_room  SaveFormat=Structure With Time  SampleTime=-1
  tag scope: T_sim=global
  wires:
  [P_room] -> Scope2/3, To Workspace2/1  "Pow"
  [V_room_ref] -> Square/1, Mux3/1  "ref"
  Mux3/1 -> Scope2/2, To Workspace1/1  "V"
  [V_room] -> Mux3/2  "real"
  [T_room] -> Sum1/1  "real"
  Constant2/1 -> Sum2/2
  Sum2/1 -> Sum/1, [T_sim]  "sim"
  Square/1 -> Gain/1
  Gain/1 -> Discrete State-Space1/1
  Discrete State-Space1/1 -> Sum2/1
  Mux1/1 -> To Workspace/1, Scope2/1
  Sum/1 -> Mux1/1
  [Temp_ref] -> Mux1/3  "ref"
  Sum1/1 -> Mux1/2
  Constant/1 -> Sum1/2, Sum/2

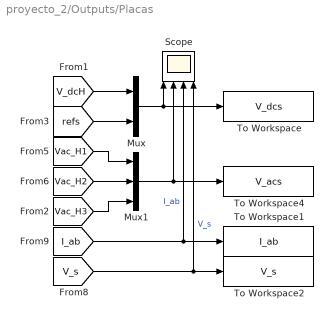
== system proyecto_2/Outputs/Placas ==
  Mux : Mux  Inputs=2
  Mux1 : Mux  Inputs=3
  Scope : Scope  NumInputPorts=4
  To Workspace : ToWorkspace  VariableName=V_dcs  SaveFormat=Structure With Time  SampleTime=-1
  To Workspace1 : ToWorkspace  VariableName=I_ab  SaveFormat=Structure With Time  SampleTime=-1
  To Workspace2 : ToWorkspace  VariableName=V_s  SaveFormat=Structure With Time  SampleTime=-1
  To Workspace4 : ToWorkspace  VariableName=V_acs  SaveFormat=Structure With Time  SampleTime=-1
  wires:
  [Vac_H2] -> Mux1/2
  [Vac_H1] -> Mux1/1
  [V_s] -> Scope/4, To Workspace2/1  "V_s"
  [refs] -> Mux/2
  [V_dcH] -> Mux/1
  Mux/1 -> Scope/1, To Workspace/1
  [Vac_H3] -> Mux1/3
  Mux1/1 -> Scope/2, To Workspace4/1
  [I_ab] -> Scope/3, To Workspace1/1  "I_ab"

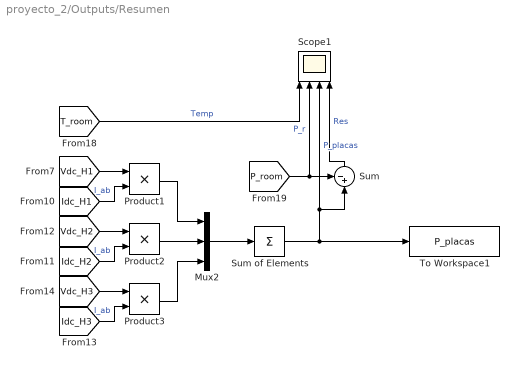
== system proyecto_2/Outputs/Resumen ==
  Mux2 : Mux  Inputs=3
  Product1 : Product
  Product2 : Product
  Product3 : Product
  Scope1 : Scope  NumInputPorts=4
  Sum : Sum  Inputs=-+|
  Sum of Elements : Sum  Inputs=+
  To Workspace1 : ToWorkspace  VariableName=P_placas  SaveFormat=Structure With Time  SampleTime=-1
  wires:
  [Vdc_H3] -> Product3/1
  [Idc_H1] -> Product1/2  "I_ab"
  Product1/1 -> Mux2/1
  [Idc_H3] -> Product3/2  "I_ab"
  Product3/1 -> Mux2/3
  [P_room] -> Sum/1, Scope1/2  "P_r"
  Product2/1 -> Mux2/2
  [Vdc_H1] -> Product1/1
  Sum of Elements/1 -> To Workspace1/1, Sum/2, Scope1/3  "P_placas"
  [Vdc_H2] -> Product2/1
  Sum/1 -> Scope1/4  "Res"
  [T_room] -> Scope1/1  "Temp"
  [Idc_H2] -> Product2/2  "I_ab"
  Mux2/1 -> Sum of Elements/1

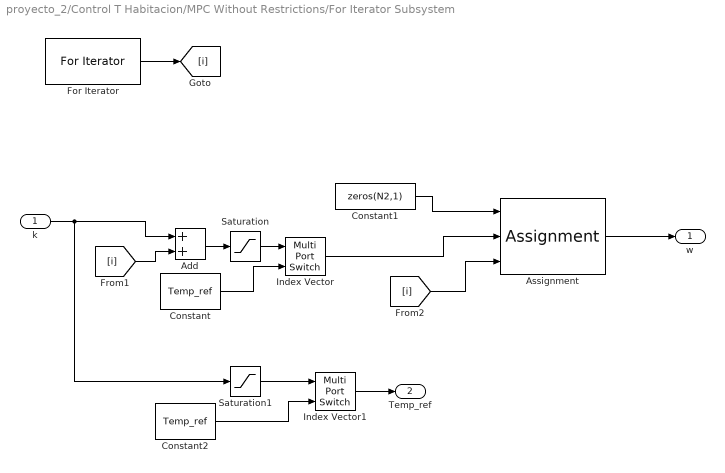
== system proyecto_2/Control T Habitacion/MPC Without Restrictions/For Iterator Subsystem ==
  k : Inport
  Add : Sum
  Assignment : Assignment  IndexMode=Zero-based  DiagnosticForDimensions=Warning  IndexOptions=Index vector (port)  Indices=1  OutputSizes=1
  Constant : Constant  Value=Temp_ref
  Constant1 : Constant  Value=zeros(N2,1)
  Constant2 : Constant  Value=Temp_ref
  For Iterator : ForIterator  IterationLimit=N2  IndexMode=Zero-based
  Index Vector : MultiPortSwitch  DataPortOrder=Zero-based contiguous  Inputs=1  zeroidx=on
  Index Vector1 : MultiPortSwitch  DataPortOrder=Zero-based contiguous  Inputs=1  zeroidx=on
  Saturation : Saturate  UpperLimit=(Tsim/T_pred)-1  LowerLimit=0
  Saturation1 : Saturate  UpperLimit=(Tsim/T_pred)-1  LowerLimit=0
  w : Outport
  Temp_ref : Outport  Port=2
  wires:
  Saturation/1 -> Index Vector/1
  Constant/1 -> Index Vector/2
  For Iterator/1 -> [i]
  Add/1 -> Saturation/1
  [i] -> Add/2
  k/1 -> Saturation1/1, Add/1
  Constant1/1 -> Assignment/1
  Index Vector/1 -> Assignment/2
  Assignment/1 -> w/1
  [i] -> Assignment/3
  Constant2/1 -> Index Vector1/2
  Index Vector1/1 -> Temp_ref/1
  Saturation1/1 -> Index Vector1/1

== system proyecto_2/Control T Habitacion/MPC Without Restrictions/Time to Discrete ==
  Clock : Clock
  Gain : Gain  Gain=1/T_pred
  Round : Rounding  Operator=round
  Scope : Scope
  tag scope: k=global
  wires:
  Clock/1 -> Gain/1
  Gain/1 -> Round/1
  Round/1 -> [k], Scope/1

== system proyecto_2/H_bridge1/H_basic/Modulator2 ==
  Mux : Mux
  Restriccion : Subsystem
  Unipolar : Subsystem
  Out1 : Outport
  wires:
  Restriccion/1(Out1) -> Mux/1
  [d_1] -> Unipolar/1(Duty)
  Mux/1 -> Out1/1
  Restriccion/4(Out4) -> Mux/4
  Unipolar/1(Out1) -> Restriccion/1(In1)
  Restriccion/3(Out3) -> Mux/3
  Unipolar/2(Out2) -> Restriccion/2(In2)
  [Triag] -> Unipolar/2(Triag)
  Restriccion/2(Out2) -> Mux/2

== system proyecto_2/H_bridge2/H_basic/Modulator2 ==
  Mux : Mux
  Restriccion : Subsystem
  Transport Delay : TransportDelay  DelayTime=shift
  Unipolar : Subsystem
  Out1 : Outport
  wires:
  Restriccion/1(Out1) -> Mux/1
  [d_2] -> Unipolar/1(Duty)
  Mux/1 -> Out1/1
  Restriccion/4(Out4) -> Mux/4
  Unipolar/1(Out1) -> Restriccion/1(In1)
  Restriccion/3(Out3) -> Mux/3
  Unipolar/2(Out2) -> Restriccion/2(In2)
  Restriccion/2(Out2) -> Mux/2
  [Triag] -> Transport Delay/1
  Transport Delay/1 -> Unipolar/2(Triag)

== system proyecto_2/H_bridge3/H_basic/Modulator2 ==
  Mux : Mux
  Restriccion : Subsystem
  Transport Delay : TransportDelay  DelayTime=2*shift
  Unipolar : Subsystem
  Out1 : Outport
  wires:
  Restriccion/1(Out1) -> Mux/1
  [d_3] -> Unipolar/1(Duty)
  Mux/1 -> Out1/1
  Restriccion/4(Out4) -> Mux/4
  Unipolar/1(Out1) -> Restriccion/1(In1)
  Restriccion/3(Out3) -> Mux/3
  Unipolar/2(Out2) -> Restriccion/2(In2)
  Restriccion/2(Out2) -> Mux/2
  [Triag] -> Transport Delay/1
  Transport Delay/1 -> Unipolar/2(Triag)

== system proyecto_2/Habitacion con calefactor/Buck-Boost/Control ==
  In1 : Inport
  Discrete PID Controller : slpidlib/PID Controller  Controller=PID  Form=Parallel  TimeDomain=Discrete-time  UseExternalTs=off  SampleTime=Ts  IntegratorMethod=Forward Euler  FilterMethod=Forward Euler  ControllerParametersSource=internal  P=2  I=10  D=0.1  UseFilter=on  N=100  TunerSelectOption=Transfer Function Based (PID Tuner App)  InitialConditionSource=internal  InitialConditionForIntegrator=0  InitialConditionForFilter=0  DifferentiatorICPrevScaledInput=0  ExternalReset=none  TrackingMode=off  Kt=1  LimitOutput=off  SatLimitsSource=internal  UpperSaturationLimit=inf  LowerSaturationLimit=-inf  LinearizeAsGain=off  AntiWindupMode=none  Kb=1  POutMin=[]  POutMax=[]  IOutMin=[]  IOutMax=[]  DOutMin=[]  DOutMax=[]  NOutMin=[]  NOutMax=[]  SumOutMin=[]  SumOutMax=[]  SaturationOutMin=[]  SaturationOutMax=[]  PParamMin=[]  PParamMax=[]  IParamMin=[]  IParamMax=[]  DParamMin=[]  DParamMax=[]  NParamMin=[]  NParamMax=[]  KbParamMin=[]  KbParamMax=[]  KtParamMin=[]  KtParamMax=[]  KbOutMin=[]  KbOutMax=[]  KtOutMin=[]  KtOutMax=[]  IntegratorOutMin=[]  IntegratorOutMax=[]  FilterOutMin=[]  FilterOutMax=[]  SumI1OutMin=[]  SumI1OutMax=[]  SumI2OutMin=[]  SumI2OutMax=[]  SumI3OutMin=[]  SumI3OutMax=[]  SumI4OutMin=[]  SumI4OutMax=[]  SumDOutMin=[]  SumDOutMax=[]  DifferentiatorOutMin=[]  DifferentiatorOutMax=[]  FilterDiffOutCoefMin=[]  FilterDiffOutCoefMax=[]  ReciprocalOutMin=[]  ReciprocalOutMax=[]  SumDenOutMin=[]  SumDenOutMax=[]  SumNumOutMin=[]  SumNumOutMax=[]  DivideOutMin=[]  DivideOutMax=[]  UdiffTsProdOutMin=[]  UdiffTsProdOutMax=[]  NTsProdOutMin=[]  NTsProdOutMax=[]  UintegralTsProdOutMin=[]  UintegralTsProdOutMax=[]  UngainTsProdOutMin=[]  UngainTsProdOutMax=[]  IntegratorContinuousStateAttributes=''  IntegratorStateMustResolveToSignalObject=off  IntegratorRTWStateStorageClass=Auto  FilterContinuousStateAttributes=''  FilterStateMustResolveToSignalObject=off  FilterRTWStateStorageClass=Auto  ParallelPVariant=InternalParameters  IdealPVariant=Disabled  IVariant=InternalParameters  DVariant=InternalParameters  IntegratorVariant=Discrete  SatVariant=Disabled  AWVariant=Passthrough  PCopyVariant=Disabled  TRVariant=Disabled  FdbkBlocksVariant=Forward  IdealPFdbkVariant=Disabled  SatFdbkVariant=Disabled  DerivativeFilterVariant=ForwardEulerFilter  NVariant=InternalParameters  NCopyVariant=Disabled  FilterICVariant=InternalICsFilter  IntegratorICVariant=InternalICs  ExternalResetVariant=Disabled  TRSumVariant=Passthrough  SumFdbkVariant=Disabled  SumVariant=Sum_PID  TsampFilterVariant=InternalTs  TsampNgainVariant=Passthrough  TsampIntegralVariant=Passthrough  ExternalSaturationOutDataTypeStr=Inherit: Same as second input
  Divide : Product  Inputs=*/
  Product : Product
  Sum : Sum  Inputs=|++
  Sum1 : Sum  Inputs=|+-
  Sum2 : Sum  Inputs=++|
  Out1 : Outport
  wires:
  [V_room] -> Sum1/2
  In1/1 -> Sum2/1, Sum1/1
  [Vdc_H4] -> Sum/2
  Sum/1 -> Divide/2
  Divide/1 -> Out1/1
  Sum2/1 -> Sum/1, Divide/1
  Discrete PID Controller/1 -> Sum2/2
  Product/1 -> Discrete PID Controller/1
  Sum1/1 -> Product/2
  [Enable] -> Product/1

== system proyecto_2/Habitacion con calefactor/Buck-Boost/Modulador ==
  In1 : Inport
  Relational Operator : RelationalOperator  OutDataTypeStr=boolean  RndMeth=Simplest
  Repeating Sequence4 : simulink/Sources/Repeating Sequence  rep_seq_t=[0 Ts/2 Ts]  rep_seq_y=[0 1 0]
  Out1 : Outport
  wires:
  In1/1 -> Relational Operator/1
  Relational Operator/1 -> Out1/1
  Repeating Sequence4/1 -> Relational Operator/2

== system proyecto_2/Habitacion con calefactor/H_bridge4/H_basic ==
  Demux : Demux
  IGBT/Diode{,1..3} (4 alike) : spsIGBTDiodeLib/IGBT//Diode  Ron=1e-3  Rs=1e5  Cs=inf  Measurements=off
  Modulator2 : Subsystem
  out + : PMIOPort  Side=Left
  out - : PMIOPort  Port=2  Side=Left
  in + : PMIOPort  Port=3  Side=Right
  in - : PMIOPort  Port=4  Side=Right
  wires:
  Demux/1 -> IGBT/Diode/1
  Demux/4 -> IGBT/Diode3/1
  Demux/2 -> IGBT/Diode2/1
  Demux/3 -> IGBT/Diode1/1
  Modulator2/1(Out1) -> Demux/1
  connections:
  IGBT/Diode2/RConn1 -- out -/RConn1 -- IGBT/Diode3/RConn1
  IGBT/Diode1/RConn1 -- in +/RConn1 -- IGBT/Diode3/LConn1
  IGBT/Diode/LConn1 -- out +/RConn1 -- IGBT/Diode1/LConn1
  IGBT/Diode/RConn1 -- in -/RConn1 -- IGBT/Diode2/LConn1
